simulink model "Flugsimulator"  (R2026a)
settings: Solver=ode45  StopTime=40  MaxStep=0.1
values from neighbouring files (symbols this model uses):
  A = [-0.1055   -0.2651   0  -0.3535 ... (first row only)    [initModel.m]
  B = [0 ... (first row only)    [initModel.m]
  C = eye(4)    [initModel.m]
  Cpid_t_D = Cpid_t.Kd    [initModel.m]
  Cpid_t_I = Cpid_t.Ki    [initModel.m]
  Cpid_t_P = Cpid_t.Kp    [initModel.m]
  Cpid_u_D = Cpid_u.Kd    [initModel.m]
  Cpid_u_I = Cpid_u.Ki    [initModel.m]
  Cpid_u_P = Cpid_u.Kp    [initModel.m]
  D = zeros(4,1)    [initModel.m]
  K = place(A,B,p)    [initModel.m]
  K_lqr = lqr(A,B,Q,R)    [initModel.m]
  L = place(A',[1 0 0 0]',observerPoles)'    [initModel.m]
  N_lqr_theta = -inv([0 0 0 1]*inv(A-B*K_lqr)*B)    [initModel.m]
  N_lqr_u = -inv([1 0 0 0]*inv(A-B*K_lqr)*B)    [initModel.m]
  N_theta = inv([0 0 0 1]*inv(B*K-A)*B)    [initModel.m]
  N_u = inv([1 0 0 0]*inv(B*K-A)*B)    [initModel.m]
  U0 = 20    [initModel.m]
libraries: slpidlib x3

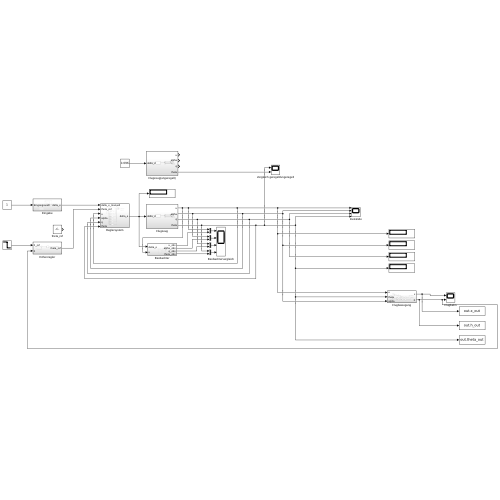
[thumbnail: Simulink's stored preview of the top-level diagram]
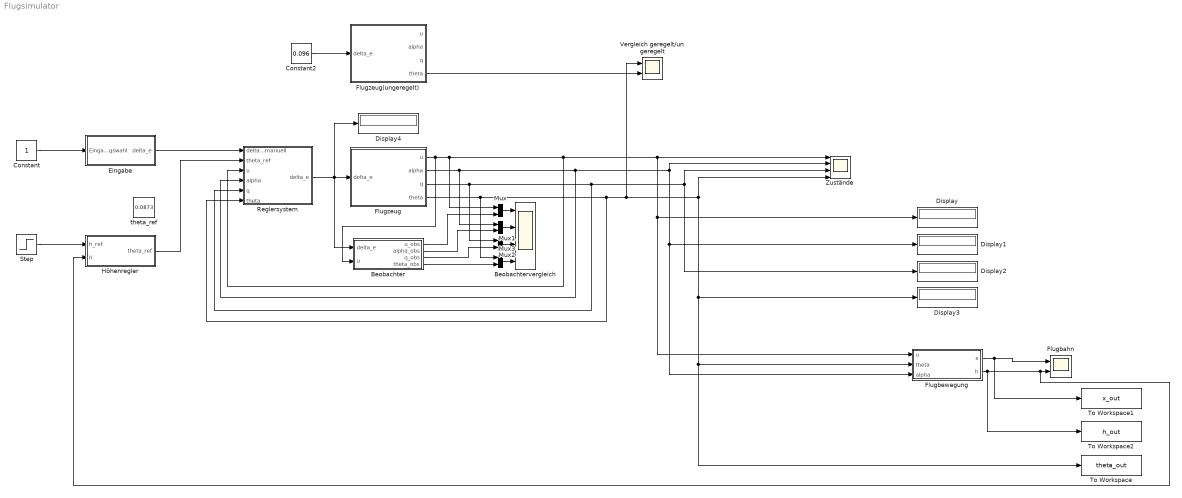
== system Flugsimulator ==
  Beobachter : Subsystem
  Beobachtervergleich : Scope  NumInputPorts=4
      settings: ActiveDisplayYMinimum=-0.0086388264736909  ActiveDisplayYMaximum=0.00095986960818787758  DataLoggingVariableName=ScopeData4
  Constant : Constant
  Constant2 : Constant  Value=0.096
  Display{,1..4} (5 alike) : Display
  Eingabe : Subsystem
  Flugbahn : Scope  NumInputPorts=2
      settings: ActiveDisplayYMinimum=-1096.1339837091905  ActiveDisplayYMaximum=2585.453560086361
  Flugbewegung : Subsystem
  Flugzeug : Subsystem
  Flugzeug(ungeregelt) : Subsystem
  Höhenregler : Subsystem
  Mux{,1..3} (4 alike) : Mux  Inputs=2
  Reglersystem : Subsystem
  Step : Step  Time=10  FinalValue=-100  SampleTime=0
  To Workspace : ToWorkspace  VariableName=theta_out  SaveFormat=Structure With Time  SampleTime=-1
  To Workspace1 : ToWorkspace  VariableName=x_out  SaveFormat=Structure With Time  SampleTime=-1
  To Workspace2 : ToWorkspace  VariableName=h_out  SaveFormat=Structure With Time  SampleTime=-1
  Vergleich geregelt/ungeregelt : Scope  NumInputPorts=2
      settings: ActiveDisplayYMinimum=-1.2578317484802715  ActiveDisplayYMaximum=0.45394678804412159  DataLoggingVariableName=ScopeData2
  Zustände : Scope  NumInputPorts=4
      settings: ActiveDisplayYMinimum=-0.38853006892856762  ActiveDisplayYMaximum=0.29324423548716205
  theta_ref : Constant  Value=0.0873
  wires:
  Flugzeug/1(u) -> Flugbewegung/1(u), Display/1, Zustände/1, Reglersystem/3(u), Mux/1, Beobachter/2(u)
  Flugzeug/4(theta) -> To Workspace/1, Flugbewegung/2(theta), Display3/1, Zustände/4, Vergleich geregelt/ungeregelt/1, Reglersystem/6(theta), Mux3/1
  Flugzeug/2(alpha) -> Flugbewegung/3(alpha), Display1/1, Zustände/2, Reglersystem/4(alpha), Mux1/1
  Flugzeug/3(q) -> Zustände/3, Display2/1, Reglersystem/5(q), Mux2/1
  Constant/1 -> Eingabe/1(Eingangswahl)
  Flugbewegung/2(h) -> To Workspace2/1, Höhenregler/2(h), Flugbahn/2
  Flugbewegung/1(x) -> To Workspace1/1, Flugbahn/1
  Eingabe/1(delta_e) -> Reglersystem/1(delta_e_manuell)
  Reglersystem/1(delta_e) -> Beobachter/1(delta_e), Display4/1, Flugzeug/1(delta_e)
  Constant2/1 -> Flugzeug(ungeregelt)/1(delta_e)
  Flugzeug(ungeregelt)/4(theta) -> Vergleich geregelt/ungeregelt/2
  Höhenregler/1(theta_ref) -> Reglersystem/2(theta_ref)
  Step/1 -> Höhenregler/1(h_ref)
  Mux/1 -> Beobachtervergleich/1
  Beobachter/1(u_obs) -> Mux/2
  Mux3/1 -> Beobachtervergleich/4
  Mux2/1 -> Beobachtervergleich/3
  Mux1/1 -> Beobachtervergleich/2
  Beobachter/2(alpha_obs) -> Mux1/2
  Beobachter/3(q_obs) -> Mux2/2
  Beobachter/4(theta_obs) -> Mux3/2

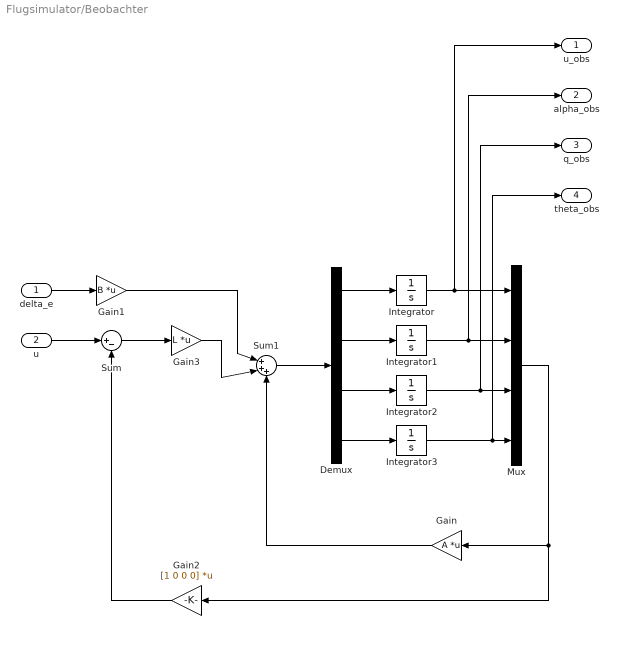
== system Flugsimulator/Beobachter ==
  delta_e : Inport
  u : Inport  Port=2
  Demux : Demux
  Gain : Gain  Gain=A  Multiplication=Matrix(K*u)
  Gain1 : Gain  Gain=B  Multiplication=Matrix(K*u)
  Gain2 : Gain  Gain=[1 0 0 0]  Multiplication=Matrix(K*u)
  Gain3 : Gain  Gain=L  Multiplication=Matrix(K*u)
  Integrator{,1..3} (4 alike) : Integrator
  Mux : Mux
  Sum : Sum  Inputs=|+-
  Sum1 : Sum  Inputs=|+++
  u_obs : Outport
  alpha_obs : Outport  Port=2
  q_obs : Outport  Port=3
  theta_obs : Outport  Port=4
  wires:
  Integrator/1 -> u_obs/1, Mux/1
  Integrator1/1 -> alpha_obs/1, Mux/2
  Integrator2/1 -> q_obs/1, Mux/3
  Integrator3/1 -> theta_obs/1, Mux/4
  Mux/1 -> Gain/1, Gain2/1
  delta_e/1 -> Gain1/1
  u/1 -> Sum/1
  Gain2/1 -> Sum/2
  Sum/1 -> Gain3/1
  Gain3/1 -> Sum1/2
  Gain1/1 -> Sum1/1
  Gain/1 -> Sum1/3
  Sum1/1 -> Demux/1
  Demux/1 -> Integrator/1
  Demux/2 -> Integrator1/1
  Demux/3 -> Integrator2/1
  Demux/4 -> Integrator3/1

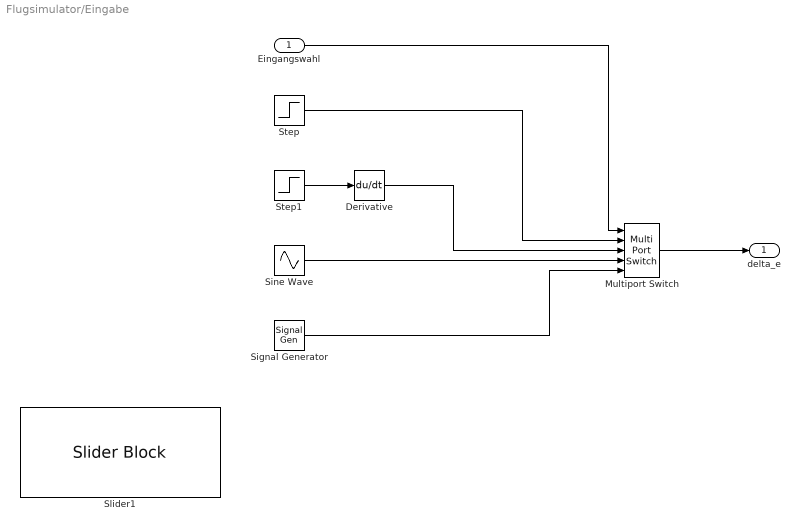
== system Flugsimulator/Eingabe ==
  Eingangswahl : Inport
  Derivative : Derivative
  Multiport Switch : MultiPortSwitch  Inputs=4  SaturateOnIntegerOverflow=off  InputSameDT=off
  Signal Generator : SignalGenerator  WaveForm=square  Amplitude=0.05  Units=rad/sec
  Sine Wave : Sin  Amplitude=0.05  Frequency=0.346079  SampleTime=0
  Slider1 : SliderBlock
  Step : Step  FinalValue=0.02  SampleTime=0
  Step1 : Step  FinalValue=0.02  SampleTime=0
  delta_e : Outport
  wires:
  Step/1 -> Multiport Switch/2
  Sine Wave/1 -> Multiport Switch/4
  Multiport Switch/1 -> delta_e/1
  Eingangswahl/1 -> Multiport Switch/1
  Signal Generator/1 -> Multiport Switch/5
  Step1/1 -> Derivative/1
  Derivative/1 -> Multiport Switch/3

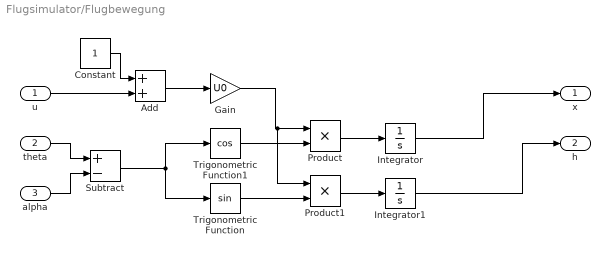
== system Flugsimulator/Flugbewegung ==
  u : Inport
  theta : Inport  Port=2
  alpha : Inport  Port=3
  Add : Sum
  Constant : Constant
  Gain : Gain  Gain=U0
  Integrator : Integrator
  Integrator1 : Integrator
  Product : Product
  Product1 : Product
  Subtract : Sum  Inputs=+-
  Trigonometric Function : Trigonometry
  Trigonometric Function1 : Trigonometry  Operator=cos
  x : Outport
  h : Outport  Port=2
  wires:
  Constant/1 -> Add/1
  u/1 -> Add/2
  Add/1 -> Gain/1
  Gain/1 -> Product1/1, Product/1
  Product/1 -> Integrator/1
  Product1/1 -> Integrator1/1
  Integrator/1 -> x/1
  Integrator1/1 -> h/1
  theta/1 -> Subtract/1
  alpha/1 -> Subtract/2
  Subtract/1 -> Trigonometric Function/1, Trigonometric Function1/1
  Trigonometric Function1/1 -> Product/2
  Trigonometric Function/1 -> Product1/2

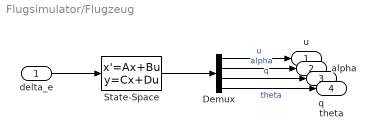
== system Flugsimulator/Flugzeug ==
  delta_e : Inport
  Demux : Demux
  State-Space : StateSpace  A=A  B=B  C=C  D=D  InitialCondition=0
  u : Outport
  alpha : Outport  Port=2
  q : Outport  Port=3
  theta : Outport  Port=4
  wires:
  State-Space/1 -> Demux/1
  Demux/2 -> alpha/1  "alpha"
  Demux/3 -> q/1  "q"
  Demux/4 -> theta/1  "theta"
  delta_e/1 -> State-Space/1
  Demux/1 -> u/1  "u"

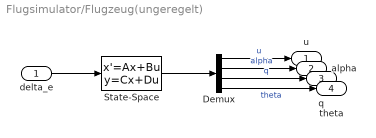
== system Flugsimulator/Flugzeug(ungeregelt) ==
  delta_e : Inport
  Demux : Demux
  State-Space : StateSpace  A=A  B=B  C=C  D=D  InitialCondition=0
  u : Outport
  alpha : Outport  Port=2
  q : Outport  Port=3
  theta : Outport  Port=4
  wires:
  State-Space/1 -> Demux/1
  Demux/2 -> alpha/1  "alpha"
  Demux/3 -> q/1  "q"
  Demux/4 -> theta/1  "theta"
  delta_e/1 -> State-Space/1
  Demux/1 -> u/1  "u"

== system Flugsimulator/Höhenregler ==
  h_ref : Inport
  h : Inport  Port=2
  PID Controller : slpidlib/PID Controller  Controller=PI  Form=Parallel  TimeDomain=Continuous-time  UseExternalTs=off  SampleTime=-1  IntegratorMethod=Forward Euler  FilterMethod=Forward Euler  ControllerParametersSource=internal  P=0.0254216893148817  I=0.000333540397006996  UseKiTs=off  D=0  UseExternalDerivativeSource=off  N=100  UseFilter=on  TunerSelectOption=Transfer Function Based (PID Tuner App)  InitialConditionSource=internal  InitialConditionForIntegrator=0  InitialConditionForFilter=0  DifferentiatorICPrevScaledInput=0  ExternalReset=none  TrackingMode=off  Kt=1  LimitOutput=on  SatLimitsSource=internal  UpperSaturationLimit=0.523599  LowerSaturationLimit=-0.523599  LinearizeAsGain=on  AntiWindupMode=external  Kb=1  LimitIntegrator=off  UpperIntegratorSaturationLimit=inf  LowerIntegratorSaturationLimit=-inf  POutMin=[]  POutMax=[]  IOutMin=[]  IOutMax=[]  DOutMin=[]  DOutMax=[]  NOutMin=[]  NOutMax=[]  SumOutMin=[]  SumOutMax=[]  SaturationOutMin=[]  SaturationOutMax=[]  PParamMin=[]  PParamMax=[]  IParamMin=[]  IParamMax=[]  DParamMin=[]  DParamMax=[]  NParamMin=[]  NParamMax=[]  KbParamMin=[]  KbParamMax=[]  KtParamMin=[]  KtParamMax=[]  KbOutMin=[]  KbOutMax=[]  KtOutMin=[]  KtOutMax=[]  IntegratorOutMin=[]  IntegratorOutMax=[]  FilterOutMin=[]  FilterOutMax=[]  SumI1OutMin=[]  SumI1OutMax=[]  SumI2OutMin=[]  SumI2OutMax=[]  SumI3OutMin=[]  SumI3OutMax=[]  SumI4OutMin=[]  SumI4OutMax=[]  SumDOutMin=[]  SumDOutMax=[]  DifferentiatorOutMin=[]  DifferentiatorOutMax=[]  FilterDiffOutCoefMin=[]  FilterDiffOutCoefMax=[]  ReciprocalOutMin=[]  ReciprocalOutMax=[]  SumDenOutMin=[]  SumDenOutMax=[]  SumNumOutMin=[]  SumNumOutMax=[]  DivideOutMin=[]  DivideOutMax=[]  UdiffTsProdOutMin=[]  UdiffTsProdOutMax=[]  NTsProdOutMin=[]  NTsProdOutMax=[]  UintegralTsProdOutMin=[]  UintegralTsProdOutMax=[]  UngainTsProdOutMin=[]  UngainTsProdOutMax=[]  ClampingZeroOutDataTypeStr=Inherit: Inherit via back propagation  ClampingZeroOutMin=[]  ClampingZeroOutMax=[]  FilterDenConstantOutDataTypeStr=Inherit: Inherit via back propagation  FilterDenConstantOutMin=[]  FilterDenConstantOutMax=[]  PCopyOutDataTypeStr=Inherit: Inherit via back propagation  PCopyOutMin=[]  PCopyOutMax=[]  NCopyOutDataTypeStr=Inherit: Inherit via back propagation  NCopyOutMin=[]  NCopyOutMax=[]  IntegratorContinuousStateAttributes=''  IntegratorStateMustResolveToSignalObject=off  IntegratorRTWStateStorageClass=Auto  FilterContinuousStateAttributes=''  FilterStateMustResolveToSignalObject=off  FilterRTWStateStorageClass=Auto  ParallelPVariant=InternalParameters  IdealPVariant=Disabled  IVariant=InternalParameters  DVariant=Disabled  IntegratorVariant=Continuous  SatVariant=Enabled  AWVariant=Passthrough  PCopyVariant=Disabled  TRVariant=Disabled  FdbkBlocksVariant=Forward  IdealPFdbkVariant=Disabled  SatFdbkVariant=Disabled  DerivativeFilterVariant=Disabled  NVariant=Disabled  NCopyVariant=Disabled_SignalSpec  FilterICVariant=Disabled  IntegratorICVariant=InternalICs  ExternalResetVariant=Disabled  TRSumVariant=Passthrough  SumFdbkVariant=Disabled  SumVariant=Sum_PI  TsampFilterVariant=InternalTs  TsampNgainVariant=Passthrough  TsampIntegralVariant=Disabled_SignalSpec  ExternalSaturationOutDataTypeStr=Inherit: Same as second input  DerivativeSourceVariant=Disabled  PreIntVariant=ExternalPreInt
  Sum : Sum  Inputs=|+-
  theta_ref : Outport
  wires:
  h_ref/1 -> Sum/1
  h/1 -> Sum/2
  Sum/1 -> PID Controller/1
  PID Controller/1 -> theta_ref/1

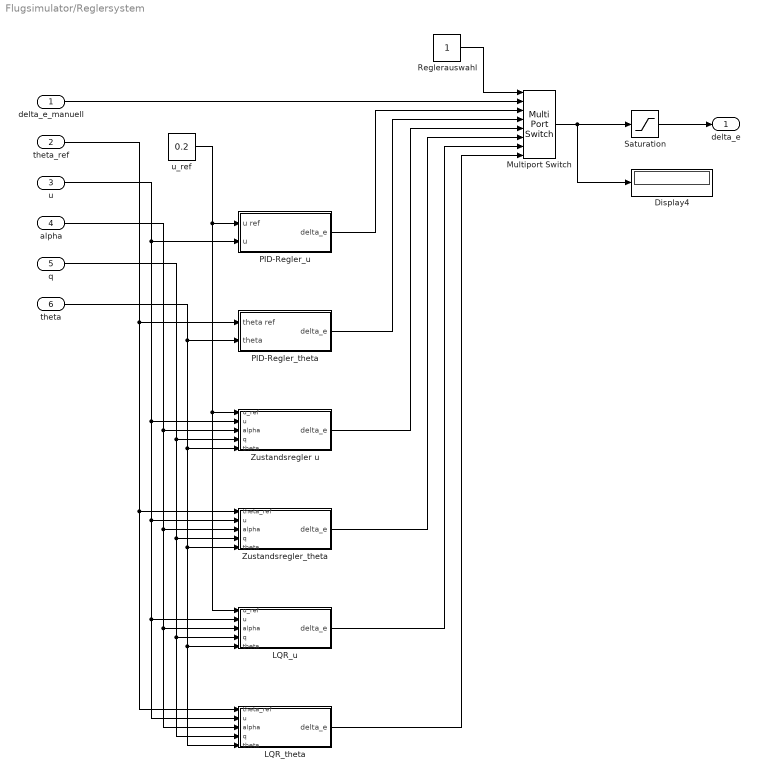
== system Flugsimulator/Reglersystem ==
  delta_e_manuell : Inport
  theta_ref : Inport  Port=2
  u : Inport  Port=3
  alpha : Inport  Port=4
  q : Inport  Port=5
  theta : Inport  Port=6
  Display4 : Display
  LQR_theta : Subsystem
  LQR_u : Subsystem
  Multiport Switch : MultiPortSwitch  Inputs=7  DiagnosticForDefault=None  SaturateOnIntegerOverflow=off  InputSameDT=off
  PID-Regler_theta : Subsystem
  PID-Regler_u : Subsystem
  Reglerauswahl : Constant
  Saturation : Saturate  UpperLimit=0.610865  LowerLimit=-0.610865
  Zustandsregler u : Subsystem
  Zustandsregler_theta : Subsystem
  u_ref : Constant  Value=0.2
  delta_e : Outport
  wires:
  delta_e_manuell/1 -> Multiport Switch/2
  Multiport Switch/1 -> Saturation/1, Display4/1
  Reglerauswahl/1 -> Multiport Switch/1
  theta_ref/1 -> PID-Regler_theta/1(theta ref), Zustandsregler_theta/1(theta_ref), LQR_theta/1(theta_ref)
  theta/1 -> LQR_u/5(theta), LQR_theta/5(theta), Zustandsregler_theta/5(theta), Zustandsregler u/5(theta), PID-Regler_theta/2(theta)
  u/1 -> PID-Regler_u/2(u), Zustandsregler u/2(u), Zustandsregler_theta/2(u), LQR_u/2(u), LQR_theta/2(u)
  u_ref/1 -> LQR_u/1(u_ref), Zustandsregler u/1(u_ref), PID-Regler_u/1(u ref)
  alpha/1 -> Zustandsregler u/3(alpha), Zustandsregler_theta/3(alpha), LQR_u/3(alpha), LQR_theta/3(alpha)
  q/1 -> LQR_theta/4(q), LQR_u/4(q), Zustandsregler_theta/4(q), Zustandsregler u/4(q)
  Zustandsregler u/1(delta_e) -> Multiport Switch/5
  Saturation/1 -> delta_e/1
  Zustandsregler_theta/1(delta_e) -> Multiport Switch/6
  LQR_u/1(delta_e) -> Multiport Switch/7
  LQR_theta/1(delta_e) -> Multiport Switch/8
  PID-Regler_u/1(delta_e) -> Multiport Switch/3
  PID-Regler_theta/1(delta_e) -> Multiport Switch/4

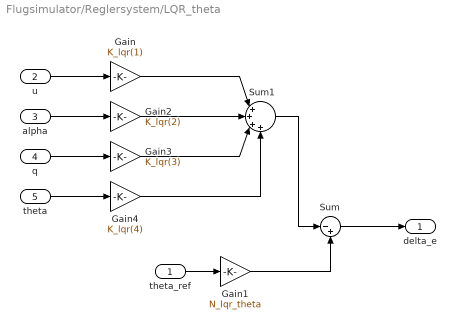
== system Flugsimulator/Reglersystem/LQR_theta ==
  theta_ref : Inport
  u : Inport  Port=2
  alpha : Inport  Port=3
  q : Inport  Port=4
  theta : Inport  Port=5
  Gain : Gain  Gain=K_lqr(1)
  Gain1 : Gain  Gain=N_lqr_theta
  Gain2 : Gain  Gain=K_lqr(2)
  Gain3 : Gain  Gain=K_lqr(3)
  Gain4 : Gain  Gain=K_lqr(4)
  Sum : Sum  Inputs=|-+
  Sum1 : Sum  Inputs=|++++
  delta_e : Outport
  wires:
  Sum/1 -> delta_e/1
  theta_ref/1 -> Gain1/1
  Gain1/1 -> Sum/2
  u/1 -> Gain/1
  alpha/1 -> Gain2/1
  q/1 -> Gain3/1
  theta/1 -> Gain4/1
  Gain/1 -> Sum1/1
  Gain2/1 -> Sum1/2
  Gain3/1 -> Sum1/3
  Gain4/1 -> Sum1/4
  Sum1/1 -> Sum/1

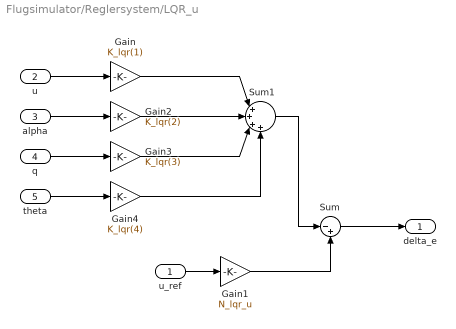
== system Flugsimulator/Reglersystem/LQR_u ==
  u_ref : Inport
  u : Inport  Port=2
  alpha : Inport  Port=3
  q : Inport  Port=4
  theta : Inport  Port=5
  Gain : Gain  Gain=K_lqr(1)
  Gain1 : Gain  Gain=N_lqr_u
  Gain2 : Gain  Gain=K_lqr(2)
  Gain3 : Gain  Gain=K_lqr(3)
  Gain4 : Gain  Gain=K_lqr(4)
  Sum : Sum  Inputs=|-+
  Sum1 : Sum  Inputs=|++++
  delta_e : Outport
  wires:
  Sum/1 -> delta_e/1
  u_ref/1 -> Gain1/1
  Gain1/1 -> Sum/2
  u/1 -> Gain/1
  alpha/1 -> Gain2/1
  q/1 -> Gain3/1
  theta/1 -> Gain4/1
  Gain/1 -> Sum1/1
  Gain2/1 -> Sum1/2
  Gain3/1 -> Sum1/3
  Gain4/1 -> Sum1/4
  Sum1/1 -> Sum/1

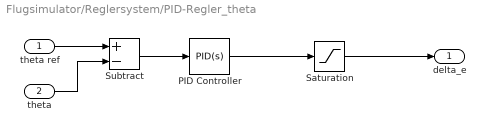
== system Flugsimulator/Reglersystem/PID-Regler_theta ==
  theta ref : Inport
  theta : Inport  Port=2
  PID Controller : slpidlib/PID Controller  Controller=PID  Form=Parallel  TimeDomain=Continuous-time  UseExternalTs=off  SampleTime=-1  IntegratorMethod=Forward Euler  FilterMethod=Forward Euler  ControllerParametersSource=internal  P=Cpid_t_P  I=Cpid_t_I  UseKiTs=off  D=Cpid_t_D  UseExternalDerivativeSource=off  N=100  UseFilter=on  TunerSelectOption=Transfer Function Based (PID Tuner App)  InitialConditionSource=internal  InitialConditionForIntegrator=0  InitialConditionForFilter=0  DifferentiatorICPrevScaledInput=0  ExternalReset=none  TrackingMode=off  Kt=1  LimitOutput=off  SatLimitsSource=internal  UpperSaturationLimit=inf  LowerSaturationLimit=-inf  LinearizeAsGain=on  AntiWindupMode=none  Kb=1  LimitIntegrator=off  UpperIntegratorSaturationLimit=inf  LowerIntegratorSaturationLimit=-inf  POutMin=[]  POutMax=[]  IOutMin=[]  IOutMax=[]  DOutMin=[]  DOutMax=[]  NOutMin=[]  NOutMax=[]  SumOutMin=[]  SumOutMax=[]  SaturationOutMin=[]  SaturationOutMax=[]  PParamMin=[]  PParamMax=[]  IParamMin=[]  IParamMax=[]  DParamMin=[]  DParamMax=[]  NParamMin=[]  NParamMax=[]  KbParamMin=[]  KbParamMax=[]  KtParamMin=[]  KtParamMax=[]  KbOutMin=[]  KbOutMax=[]  KtOutMin=[]  KtOutMax=[]  IntegratorOutMin=[]  IntegratorOutMax=[]  FilterOutMin=[]  FilterOutMax=[]  SumI1OutMin=[]  SumI1OutMax=[]  SumI2OutMin=[]  SumI2OutMax=[]  SumI3OutMin=[]  SumI3OutMax=[]  SumI4OutMin=[]  SumI4OutMax=[]  SumDOutMin=[]  SumDOutMax=[]  DifferentiatorOutMin=[]  DifferentiatorOutMax=[]  FilterDiffOutCoefMin=[]  FilterDiffOutCoefMax=[]  ReciprocalOutMin=[]  ReciprocalOutMax=[]  SumDenOutMin=[]  SumDenOutMax=[]  SumNumOutMin=[]  SumNumOutMax=[]  DivideOutMin=[]  DivideOutMax=[]  UdiffTsProdOutMin=[]  UdiffTsProdOutMax=[]  NTsProdOutMin=[]  NTsProdOutMax=[]  UintegralTsProdOutMin=[]  UintegralTsProdOutMax=[]  UngainTsProdOutMin=[]  UngainTsProdOutMax=[]  ClampingZeroOutDataTypeStr=Inherit: Inherit via back propagation  ClampingZeroOutMin=[]  ClampingZeroOutMax=[]  FilterDenConstantOutDataTypeStr=Inherit: Inherit via back propagation  FilterDenConstantOutMin=[]  FilterDenConstantOutMax=[]  PCopyOutDataTypeStr=Inherit: Inherit via back propagation  PCopyOutMin=[]  PCopyOutMax=[]  NCopyOutDataTypeStr=Inherit: Inherit via back propagation  NCopyOutMin=[]  NCopyOutMax=[]  IntegratorContinuousStateAttributes=''  IntegratorStateMustResolveToSignalObject=off  IntegratorRTWStateStorageClass=Auto  FilterContinuousStateAttributes=''  FilterStateMustResolveToSignalObject=off  FilterRTWStateStorageClass=Auto  ParallelPVariant=InternalParameters  IdealPVariant=Disabled  IVariant=InternalParameters  DVariant=InternalParameters  IntegratorVariant=Continuous  SatVariant=Disabled  AWVariant=Passthrough  PCopyVariant=Disabled  TRVariant=Disabled  FdbkBlocksVariant=Forward  IdealPFdbkVariant=Disabled  SatFdbkVariant=Disabled  DerivativeFilterVariant=ContFilter  NVariant=InternalParameters  NCopyVariant=Disabled  FilterICVariant=InternalICsFilter  IntegratorICVariant=InternalICs  ExternalResetVariant=Disabled  TRSumVariant=Passthrough  SumFdbkVariant=Disabled  SumVariant=Sum_PID  TsampFilterVariant=InternalTs  TsampNgainVariant=Passthrough  TsampIntegralVariant=Disabled_SignalSpec  ExternalSaturationOutDataTypeStr=Inherit: Same as second input  DerivativeSourceVariant=ErrorSignal  PreIntVariant=InternalPreInt
  Saturation : Saturate  UpperLimit=0.610865  LowerLimit=-0.610865
  Subtract : Sum  Inputs=+-
  delta_e : Outport
  wires:
  theta/1 -> Subtract/2
  theta ref/1 -> Subtract/1
  Subtract/1 -> PID Controller/1
  PID Controller/1 -> Saturation/1
  Saturation/1 -> delta_e/1

== system Flugsimulator/Reglersystem/PID-Regler_u ==
  u ref : Inport
  u : Inport  Port=2
  PID Controller : slpidlib/PID Controller  Controller=PID  Form=Parallel  TimeDomain=Continuous-time  UseExternalTs=off  SampleTime=-1  IntegratorMethod=Forward Euler  FilterMethod=Forward Euler  ControllerParametersSource=internal  P=Cpid_u_P  I=Cpid_u_I  UseKiTs=off  D=Cpid_u_D  UseExternalDerivativeSource=off  N=100  UseFilter=on  TunerSelectOption=Transfer Function Based (PID Tuner App)  InitialConditionSource=internal  InitialConditionForIntegrator=0  InitialConditionForFilter=0  DifferentiatorICPrevScaledInput=0  ExternalReset=none  TrackingMode=off  Kt=1  LimitOutput=off  SatLimitsSource=internal  UpperSaturationLimit=inf  LowerSaturationLimit=-inf  LinearizeAsGain=on  AntiWindupMode=none  Kb=1  LimitIntegrator=off  UpperIntegratorSaturationLimit=inf  LowerIntegratorSaturationLimit=-inf  POutMin=[]  POutMax=[]  IOutMin=[]  IOutMax=[]  DOutMin=[]  DOutMax=[]  NOutMin=[]  NOutMax=[]  SumOutMin=[]  SumOutMax=[]  SaturationOutMin=[]  SaturationOutMax=[]  PParamMin=[]  PParamMax=[]  IParamMin=[]  IParamMax=[]  DParamMin=[]  DParamMax=[]  NParamMin=[]  NParamMax=[]  KbParamMin=[]  KbParamMax=[]  KtParamMin=[]  KtParamMax=[]  KbOutMin=[]  KbOutMax=[]  KtOutMin=[]  KtOutMax=[]  IntegratorOutMin=[]  IntegratorOutMax=[]  FilterOutMin=[]  FilterOutMax=[]  SumI1OutMin=[]  SumI1OutMax=[]  SumI2OutMin=[]  SumI2OutMax=[]  SumI3OutMin=[]  SumI3OutMax=[]  SumI4OutMin=[]  SumI4OutMax=[]  SumDOutMin=[]  SumDOutMax=[]  DifferentiatorOutMin=[]  DifferentiatorOutMax=[]  FilterDiffOutCoefMin=[]  FilterDiffOutCoefMax=[]  ReciprocalOutMin=[]  ReciprocalOutMax=[]  SumDenOutMin=[]  SumDenOutMax=[]  SumNumOutMin=[]  SumNumOutMax=[]  DivideOutMin=[]  DivideOutMax=[]  UdiffTsProdOutMin=[]  UdiffTsProdOutMax=[]  NTsProdOutMin=[]  NTsProdOutMax=[]  UintegralTsProdOutMin=[]  UintegralTsProdOutMax=[]  UngainTsProdOutMin=[]  UngainTsProdOutMax=[]  ClampingZeroOutDataTypeStr=Inherit: Inherit via back propagation  ClampingZeroOutMin=[]  ClampingZeroOutMax=[]  FilterDenConstantOutDataTypeStr=Inherit: Inherit via back propagation  FilterDenConstantOutMin=[]  FilterDenConstantOutMax=[]  PCopyOutDataTypeStr=Inherit: Inherit via back propagation  PCopyOutMin=[]  PCopyOutMax=[]  NCopyOutDataTypeStr=Inherit: Inherit via back propagation  NCopyOutMin=[]  NCopyOutMax=[]  IntegratorContinuousStateAttributes=''  IntegratorStateMustResolveToSignalObject=off  IntegratorRTWStateStorageClass=Auto  FilterContinuousStateAttributes=''  FilterStateMustResolveToSignalObject=off  FilterRTWStateStorageClass=Auto  ParallelPVariant=InternalParameters  IdealPVariant=Disabled  IVariant=InternalParameters  DVariant=InternalParameters  IntegratorVariant=Continuous  SatVariant=Disabled  AWVariant=Passthrough  PCopyVariant=Disabled  TRVariant=Disabled  FdbkBlocksVariant=Forward  IdealPFdbkVariant=Disabled  SatFdbkVariant=Disabled  DerivativeFilterVariant=ContFilter  NVariant=InternalParameters  NCopyVariant=Disabled  FilterICVariant=InternalICsFilter  IntegratorICVariant=InternalICs  ExternalResetVariant=Disabled  TRSumVariant=Passthrough  SumFdbkVariant=Disabled  SumVariant=Sum_PID  TsampFilterVariant=InternalTs  TsampNgainVariant=Passthrough  TsampIntegralVariant=Disabled_SignalSpec  ExternalSaturationOutDataTypeStr=Inherit: Same as second input  DerivativeSourceVariant=ErrorSignal  PreIntVariant=InternalPreInt
  Saturation : Saturate  UpperLimit=0.610865  LowerLimit=-0.610865
  Subtract : Sum  Inputs=+-
  delta_e : Outport
  wires:
  u/1 -> Subtract/2
  u ref/1 -> Subtract/1
  Subtract/1 -> PID Controller/1
  PID Controller/1 -> Saturation/1
  Saturation/1 -> delta_e/1

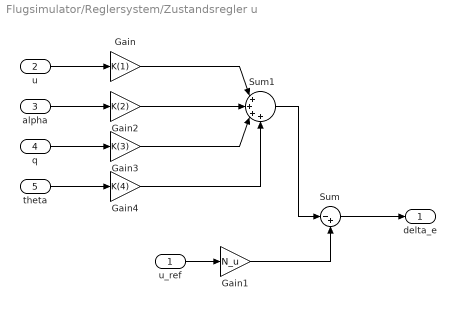
== system Flugsimulator/Reglersystem/Zustandsregler u ==
  u_ref : Inport
  u : Inport  Port=2
  alpha : Inport  Port=3
  q : Inport  Port=4
  theta : Inport  Port=5
  Gain : Gain  Gain=K(1)
  Gain1 : Gain  Gain=N_u
  Gain2 : Gain  Gain=K(2)
  Gain3 : Gain  Gain=K(3)
  Gain4 : Gain  Gain=K(4)
  Sum : Sum  Inputs=|-+
  Sum1 : Sum  Inputs=|++++
  delta_e : Outport
  wires:
  Sum/1 -> delta_e/1
  u_ref/1 -> Gain1/1
  Gain1/1 -> Sum/2
  u/1 -> Gain/1
  alpha/1 -> Gain2/1
  q/1 -> Gain3/1
  theta/1 -> Gain4/1
  Gain/1 -> Sum1/1
  Gain2/1 -> Sum1/2
  Gain3/1 -> Sum1/3
  Gain4/1 -> Sum1/4
  Sum1/1 -> Sum/1

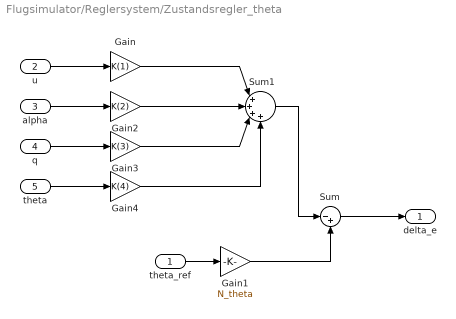
== system Flugsimulator/Reglersystem/Zustandsregler_theta ==
  theta_ref : Inport
  u : Inport  Port=2
  alpha : Inport  Port=3
  q : Inport  Port=4
  theta : Inport  Port=5
  Gain : Gain  Gain=K(1)
  Gain1 : Gain  Gain=N_theta
  Gain2 : Gain  Gain=K(2)
  Gain3 : Gain  Gain=K(3)
  Gain4 : Gain  Gain=K(4)
  Sum : Sum  Inputs=|-+
  Sum1 : Sum  Inputs=|++++
  delta_e : Outport
  wires:
  Sum/1 -> delta_e/1
  theta_ref/1 -> Gain1/1
  Gain1/1 -> Sum/2
  u/1 -> Gain/1
  alpha/1 -> Gain2/1
  q/1 -> Gain3/1
  theta/1 -> Gain4/1
  Gain/1 -> Sum1/1
  Gain2/1 -> Sum1/2
  Gain3/1 -> Sum1/3
  Gain4/1 -> Sum1/4
  Sum1/1 -> Sum/1
